simulink model "CPA1"  (R2012b)
settings: Solver=ode1  StartTime=0.0  StopTime=5  FixedStep=0.05  RelTol=1e-3
libraries: opclib x5
settings Model: Creator=Leonardo  LastModifiedBy=Josias
settings DataIOCC: SignalLoggingSaveFormat=ModelDataLogs
settings OptimizationCC: ExpressionDepthLimit=128
settings DebuggingCC: UnderspecifiedInitializationDetection=Simplified  MultiTaskDSMMsg=warning  MultiTaskCondExecSysMsg=none  StateNameClashWarn=none  StrictBusMsg=None
settings RTWCC: IncludeERTFirstTime=on
settings CodeAppCC: CustomSymbolStrType=$N$R$M_T  InternalIdentifier=Shortened
settings GRTTargetCC: CodeReplacementLibrary=None  CPPClassGenCompliant=on

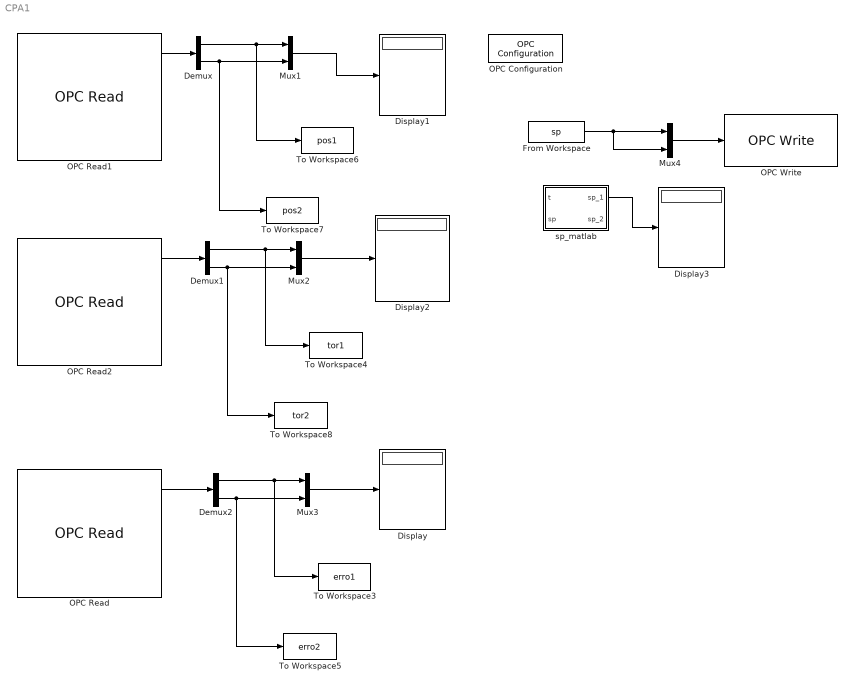
== system CPA1 ==
  Demux : Demux  Outputs=2
  Demux1 : Demux  Outputs=2
  Demux2 : Demux  Outputs=2
  Display{,1..3} (4 alike) : Display
  From Workspace : FromWorkspace  VariableName=sp  SampleTime=0
  Mux{1..4} (4 alike) : Mux  Inputs=2
  OPC Configuration : opclib/OPC Configuration  opcServers=localhost/ElipseSCADA.OPCSvr.1/10  errMissingItems=Error  errReadWrite=Warn  errShutdown=Error  errRTViolation=Warn  rtEnable=on  speedup=1  showLatency=off  beingUsed=on
  OPC Read : opclib/OPC Read  serverHost=localhost  serverID=ElipseSCADA.OPCSvr.1  itemIDs=Tags.Erro_J1, Tags.Erro_J2  readMode=Synchronous (cache)  dataType=double  updateRate=0.05  showQual=on  showTS=on  tsMode=Seconds since start
  OPC Read1 : opclib/OPC Read  serverHost=localhost  serverID=ElipseSCADA.OPCSvr.1  itemIDs=Tags.posição1, Tags.Posição2  readMode=Synchronous (cache)  dataType=double  updateRate=0.05  showQual=on  showTS=on  tsMode=Seconds since start
  OPC Read2 : opclib/OPC Read  serverHost=localhost  serverID=ElipseSCADA.OPCSvr.1  itemIDs=Tags.sinal_junta_1, Tags.sinal_junta_2  readMode=Synchronous (cache)  dataType=double  updateRate=0.05  showQual=on  showTS=on  tsMode=Seconds since start
  OPC Write : opclib/OPC Write  serverHost=localhost  serverID=ElipseSCADA.OPCSvr.1  itemIDs=Tags.setpoint_teta_1, Tags.setpoint_teta_2  writeMode=Synchronous  updateRate=0.05
  To Workspace3 : ToWorkspace  VariableName=erro1  SampleTime=-1
  To Workspace4 : ToWorkspace  VariableName=tor1  SampleTime=-1
  To Workspace5 : ToWorkspace  VariableName=erro2  SampleTime=-1
  To Workspace6 : ToWorkspace  VariableName=pos1  SampleTime=-1
  To Workspace7 : ToWorkspace  VariableName=pos2  SampleTime=-1
  To Workspace8 : ToWorkspace  VariableName=tor2  SampleTime=-1
  sp_matlab : MATLAB Function  TreatAsAtomicUnit=on
  wires:
  Demux/2 -> To Workspace7/1, Mux1/2
  Demux/1 -> To Workspace6/1, Mux1/1
  OPC Read1/1 -> Demux/1
  Demux1/2 -> To Workspace8/1, Mux2/2
  Demux1/1 -> To Workspace4/1, Mux2/1
  OPC Read2/1 -> Demux1/1
  Mux2/1 -> Display2/1
  Demux2/2 -> To Workspace5/1, Mux3/2
  Demux2/1 -> To Workspace3/1, Mux3/1
  OPC Read/1 -> Demux2/1
  Mux3/1 -> Display/1
  Mux1/1 -> Display1/1
  From Workspace/1 -> Mux4/2, Mux4/1
  Mux4/1 -> OPC Write/1
  sp_matlab/1(sp_1) -> Display3/1

== matlab function CPA1/sp_matlab ==
  data: sp_1 output; t input; sp_2 output; sp input
function [sp_1, sp_2] = fcn(t, sp)
%#codegen
sp;

y =[sp_1 sp_2];
